simulink model "ProjetPart1"  (R2021b)
settings: Solver=VariableStepAuto  StartTime=0.0  StopTime=inf  RelTol=1e-3
libraries: dspspect3 x1, dspvision x1, dspobslib x1
settings Model: Creator=coren  LastModifiedBy=coren

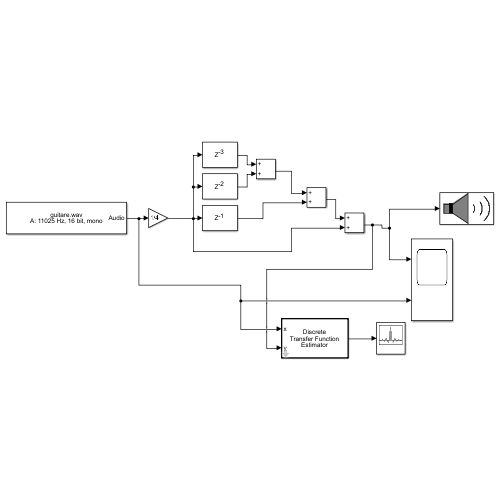
[thumbnail: Simulink's stored preview of the top-level diagram]
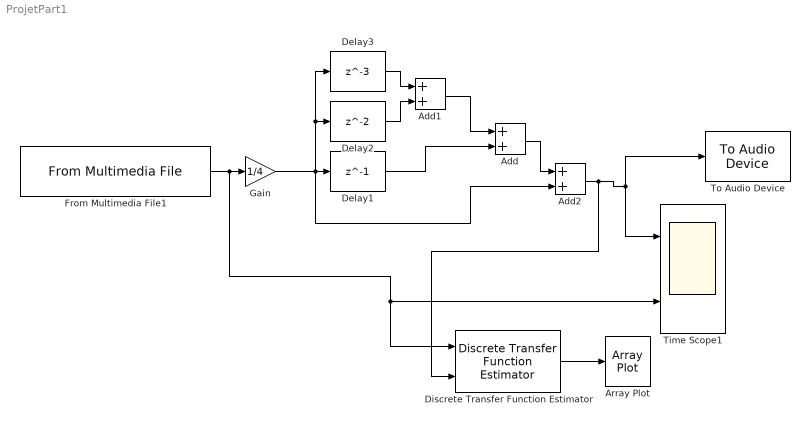
== system ProjetPart1 ==
  Add : Sum
  Add1 : Sum
  Add2 : Sum
  Array Plot : ArrayPlot
  Delay1 : Delay  DelayLength=1  DelayLengthUpperLimit=5000  InputProcessing=Columns as channels (frame based)
  Delay2 : Delay  DelayLengthUpperLimit=5000  InputProcessing=Columns as channels (frame based)
  Delay3 : Delay  DelayLength=3  DelayLengthUpperLimit=5000  InputProcessing=Columns as channels (frame based)
  Discrete Transfer Function Estimator : dspspect3/Discrete Transfer Function Estimator  WindowMode=Specify on dialog  WindowLength=1024  Overlap=50  AveragingMethod=Running  ForgettingFactorPort=off  ForgettingFactor=0.9  SpectralAverages=100  FFTLengthSource=Auto  FFTLength=128  Window=Hann  SidelobeAttenuation=60  FrequencyRange=One-sided  OutputCoherence=off  SimulateUsing=Code generation
      settings: SourceProductBaseCode=DS
  From Multimedia File1 : dspvision/From Multimedia File  inputFilename=C:\Users\coren\Documents\MATLAB\Traitement Images et Son 3E105\Projet Son\guitare.wav  readRange=[1 Inf]  loop=on  numPlays=inf  outputStreams=Audio only  videoDataType=single  audioDataType=double  inheritSampleTime=on  userDefinedSampleTime=1/30  noAudioOutput=off  isIntensityVideo=off  fourcc=RGB  colorVideoFormat=Separate color signals  outputEOF=off  dataOrg=Column-major  audioFrameSize=1024  computeAudioFrameSize=off  outSamplingMode=Sample based
  Gain : Gain  Gain=1/4
  Time Scope1 : Scope  NumInputPorts=2
  To Audio Device : dspobslib/To Audio Device  deviceName=Default  inheritSampleRate=on  sampleRate=44100  deviceDatatype=Determine from input data type  autoBufferSize=on  bufferSize=4096  queueDuration=1.0  defaultOutputChannelMapping=on  outputChannelMapping=1:2  outputNumUnderrunSamples=off
      settings: SourceProductBaseCode=DS
  wires:
  Gain/1 -> Delay3/1, Delay2/1, Delay1/1, Add2/2
  From Multimedia File1/1 -> Discrete Transfer Function Estimator/1, Time Scope1/2, Gain/1
  Delay1/1 -> Add/2
  Delay3/1 -> Add1/1
  Delay2/1 -> Add1/2
  Add1/1 -> Add/1
  Add/1 -> Add2/1
  Add2/1 -> Discrete Transfer Function Estimator/2, To Audio Device/1, Time Scope1/1
  Discrete Transfer Function Estimator/1 -> Array Plot/1
